simulink model "ex_3"  (R2016a)
settings: Solver=VariableStepAuto  StartTime=0.0  StopTime=10.0  RelTol=1e-3
settings Model: Creator=Linstar  LastModifiedBy=Linstar

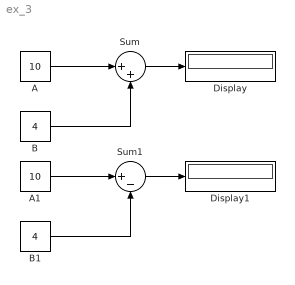
== system ex_3 ==
  A : Constant  Value=10
  A1 : Constant  Value=10
  B : Constant  Value=4
  B1 : Constant  Value=4
  Display : Display
  Display1 : Display
  Sum : Sum  Inputs=|++
  Sum1 : Sum  Inputs=|+-
  wires:
  B/1 -> Sum/2
  A/1 -> Sum/1
  Sum/1 -> Display/1
  B1/1 -> Sum1/2
  A1/1 -> Sum1/1
  Sum1/1 -> Display1/1
